simulink model "dts_adc1"  (R2023b)
settings: Solver=VariableStepAuto  StartTime=0.0  StopTime=3*DF/Fs  MaxStep=10/12e6  MinStep=1/12e6  RelTol=1e-9  AbsTol=1e-9  EnableMultiTasking=on
model workspace (MAT data in the model file):
  Q = 1.6e-19
  k = 1.38e-23
  m = 4
  p = 8
values from neighbouring files (symbols this model uses):
  a = 4.32    [ADC_data2.m]    (also in ADC_filter_data.mat)
  DF = 512    [ADC_data2.m]    (also in ADC_filter_data.mat)
  Fs = 1e+06    (= 1000000)    [ADC_data2.m]    (also in ADC_filter_data.mat)
  T = temp + 273.15    [ADC_data2.m]    (also in ADC_filter_data.mat = 428.15)
  vctat = -VCTAT(i)    [ADC_data2.m]    (also in ADC_filter_data.mat = -0.648)
  vn = 10e-6    (= 1e-05)    [ADC_data2.m]    (also in ADC_filter_data.mat)
  vos = 0    [ADC_data2.m]    (also in ADC_filter_data.mat)
  vptat = VPTAT(i)    [ADC_data2.m]    (also in ADC_filter_data.mat = 0.692)
undefined symbols (not defined in the file or in its folder): Nsamples, OSR
libraries: dspstat3 x2, dspsigops x2
settings Model: Creator=amyles  LastModifiedBy=SinhaAd
settings SolverCC: InitialStep=0  AlgebraicLoopSolver=TrustRegion
settings DataIOCC: LimitDataPoints=on  MaxDataPoints=50000  SaveFormat=Array  ReturnWorkspaceOutputs=off  Refine=10
settings OptimizationCC: DefaultParameterBehavior=Inlined  ExpressionDepthLimit=2147483647  LifeSpan=inf
settings DebuggingCC: SolverPrmCheckMsg=warning  FcnCallInpInsideContextMsg=warning  UnconnectedInputMsg=warning  UnconnectedOutputMsg=warning  UnconnectedLineMsg=warning  StateNameClashWarn=warning  StrictBusMsg=ErrorOnBusTreatedAsVector  SFUnexpectedBacktrackingDiag=warning  SFNoUnconditionalDefaultTransitionDiag=warning  SFExecutionAtInitializationDiag=none  ArithmeticOperatorsInVariantConditions=warning
settings HardwareCC: ProdBitPerPointer=32  ProdBitPerSizeT=32  ProdBitPerPtrDiffT=32  ProdLargestAtomicFloat=None  ProdIntDivRoundTo=Undefined  ProdEndianess=Unspecified  ProdWordSize=32  ProdHWDeviceType=32-bit Generic
settings ModelReferenceCC: EnableRefExpFcnMdlSchedulingChecks=on  ModelReferenceNumInstancesAllowed=Single  PropagateSignalLabelsOutOfModel=off
settings SFSimCC: SimUseLocalCustomCode=off  CustomCodeUndefinedFunction=UseInterfaceOnly
settings RTWCC: RTWUseLocalCustomCode=off  DLArmComputeVersion=19.05
settings CodeAppCC: StateflowObjectComments=on
settings GRTTargetCC: TargetLangStandard=C89/C90 (ANSI)  CombineOutputUpdateFcns=off  GRTInterface=on
settings ConfigComp: CovMetricSettings=dw  CovSaveCumulativeToWorkspaceVar=on  CovSaveSingleToWorkspaceVar=on  CovExternalEMLEnable=off

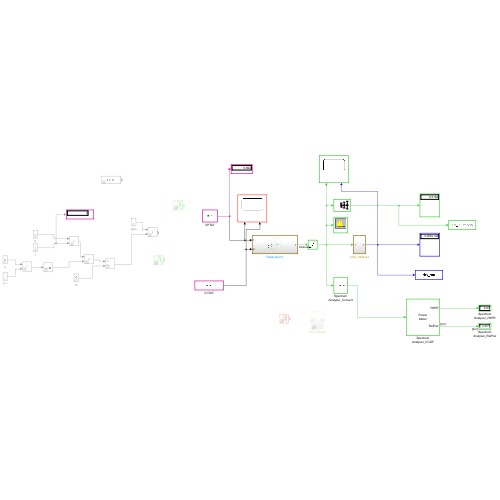
[thumbnail: Simulink's stored preview of the top-level diagram]
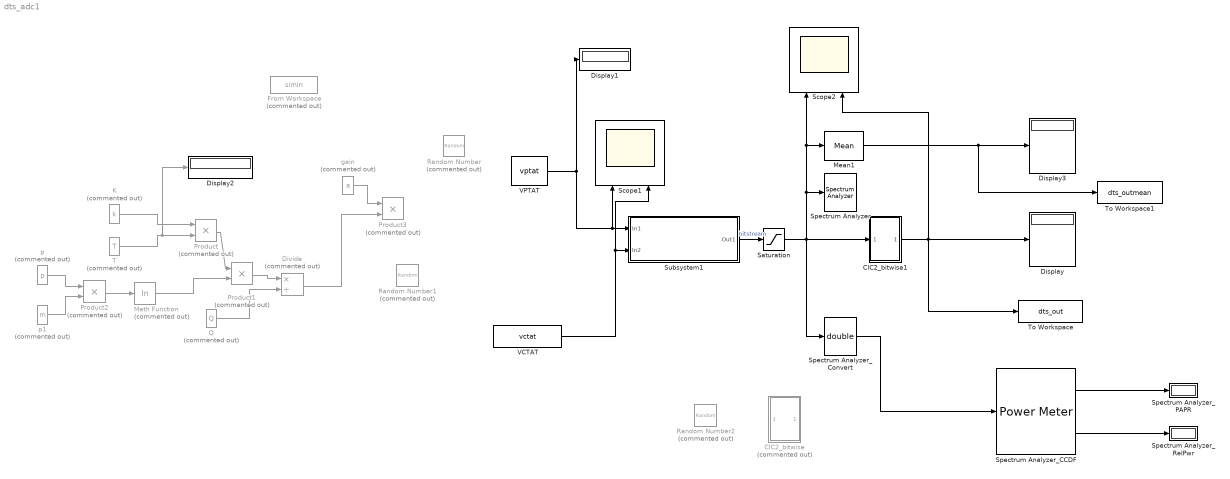
== system dts_adc1 ==
  CIC2_bitwise : Subsystem  Commented=on
  CIC2_bitwise1 : Subsystem
  Display{,1..3} (4 alike) : Display
  Divide : Product  Commented=on  Inputs=*/
  From Workspace : FromWorkspace  Commented=on  VariableName=simin
  K : Constant  Commented=on  Value=k
  Math Function : Math  Commented=on  Operator=log
  Mean1 : dspstat3/Mean  run=on  reset_popup=None  directionMode=Entire input  dimension=1  roiEnable=off  roiType=Rectangles  roiPortion=Entire ROI  roiOutput=Individual statistics for each ROI  roiFlag=off  roundingMode=Floor  overflowMode=off  outputDataTypeStr=Inherit: Same as accumulator  outputMin=[]  outputMax=[]  outputLastDataTypeStr=Inherit: Same as accumulator
  Product{,1..3} (4 alike) : Product  Commented=on
  Q : Constant  Commented=on  Value=Q
  Random Number : RandomNumber  Commented=on  Variance=(vn)^2  Seed=12345  SampleTime=1/(10*Fs)
  Random Number1 : RandomNumber  Commented=on  Variance=(vn)^2  SampleTime=1/(10*Fs)
  Random Number2 : RandomNumber  Commented=on  Variance=(1e-3)^2  SampleTime=1/(10*Fs)
  Saturation : Saturate  UpperLimit=1  LowerLimit=0
  Scope1 : Scope  NumInputPorts=2
  Scope2 : Scope  NumInputPorts=2
  Spectrum Analyzer : SpectrumAnalyzer  WindowPosition=[196.000000,277.000000,1278.000000,670.000000,]  Visible=on  ScopeFrameLocation=window  Method=Welch  SampleRateSource=Property  SampleRate=Fs  PlotAsTwoSidedSpectrum=off  FrequencyScale=Log  AveragingMethod=Exponential  YLimits=[-62.38980233,33.88782663]  SelectedToolstripTab=spectrumAnalyzerToolstrip.measurementsTab  DefaultConfigurationName=spbscopes.SpectrumAnalyzerBlockCfg  IsFrequencyInputMode=0  FrequencyVectorPort=0  FrequencyVectorFromPort=0  FrequencyInputRBWPort=0  FrequencyInputRBWFromPort=0
  Spectrum Analyzer_CCDF : dspstat3/Power Meter  Measurement=Peak-to-average power ratio  ReferenceLoad=1  OutputPowerUnits=dBm  WindowLength=256  OverlapLength=255  AllowArbitraryInputLength=off  ComputeCCDF=on  PowerRange=50  PowerResolution=0.1  CCDFOutput=Relative power (dB above average power)  ProbabilityVector=[ 10; 1; 0.1; 0.01; 0.001; 0.0001 ]  RelativePowerVector=[ 0; 3; 6; 9; 12 ]  ResetPort=off  SimulateUsing=Code generation
  Spectrum Analyzer_Convert : DataTypeConversion  OutDataTypeStr=double
  Spectrum Analyzer_PAPR : Display
  Spectrum Analyzer_RelPwr : Display
  Subsystem1 : Subsystem
  T : Constant  Commented=on  Value=T
  To Workspace : ToWorkspace  VariableName=dts_out  SaveFormat=Timeseries  SampleTime=-1
  To Workspace1 : ToWorkspace  VariableName=dts_outmean  SaveFormat=Timeseries  SampleTime=-1
  VCTAT : Constant  Value=vctat
  VPTAT : Constant  Value=vptat
  gain : Constant  Commented=on  Value=a
  p : Constant  Commented=on  Value=p
  p1 : Constant  Commented=on  Value=m
  wires:
  VPTAT/1 -> Scope1/1, Subsystem1/1(In1), Display1/1
  Subsystem1/1(Out1) -> Saturation/1  "bitstream"
  K/1 -> Product/1
  T/1 -> Display2/1, Product/2
  Q/1 -> Divide/2
  Product/1 -> Product1/1
  Product1/1 -> Divide/1
  Product2/1 -> Math Function/1
  p/1 -> Product2/1
  p1/1 -> Product2/2
  Math Function/1 -> Product1/2
  Divide/1 -> Product3/2
  gain/1 -> Product3/1
  Saturation/1 -> Spectrum Analyzer_Convert/1, Spectrum Analyzer/1, Mean1/1, Scope2/1, CIC2_bitwise1/1(In1)
  CIC2_bitwise1/1(Outport) -> Scope2/2, To Workspace/1, Display/1
  VCTAT/1 -> Scope1/2, Subsystem1/2(In2)
  Spectrum Analyzer_Convert/1 -> Spectrum Analyzer_CCDF/1
  Spectrum Analyzer_CCDF/1 -> Spectrum Analyzer_PAPR/1
  Spectrum Analyzer_CCDF/2 -> Spectrum Analyzer_RelPwr/1
  Mean1/1 -> To Workspace1/1, Display3/1

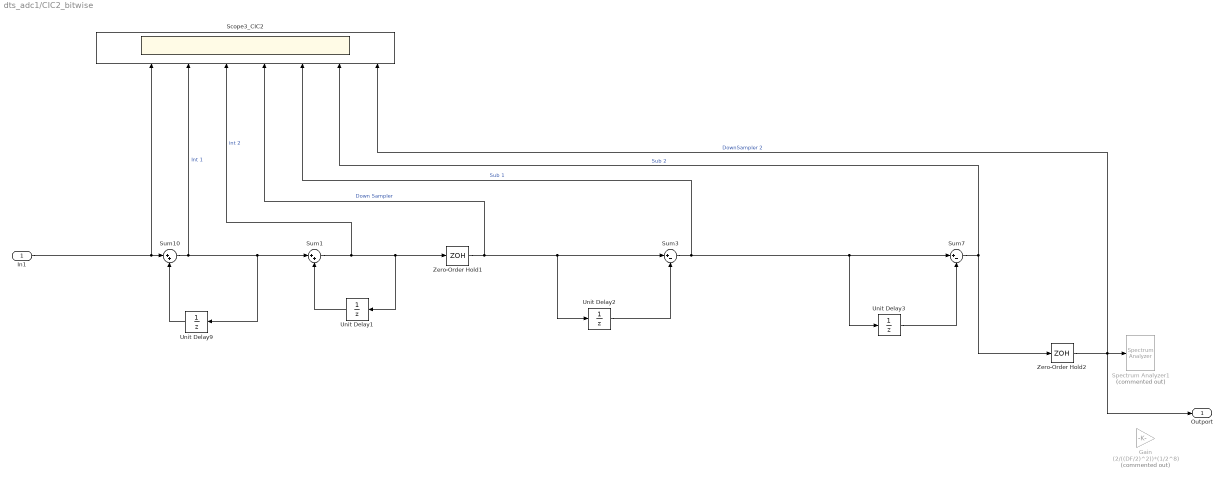
== system dts_adc1/CIC2_bitwise ==
  In1 : Inport
  Gain : Gain  Commented=on  Gain=(2/((DF/2)^2))*(1/2^8)
  Scope3_CIC2 : Scope  NumInputPorts=8
  Spectrum Analyzer1 : SpectrumAnalyzer  Commented=on  WindowPosition=[1.8 41.8 1534.4 740.8]  Method=Welch  SampleRate=5859.375  PlotAsTwoSidedSpectrum=off  AxesScaling=Manual  FrequencySpan=Start and stop frequencies  Span=(2*16*12e6)/2048  StartFrequency=0.9  StopFrequency=Fs/(2*32*OSR)  FrequencyResolutionMethod=Window length  WindowLength=(Nsamples)/(OSR)  AveragingMethod=Exponential  YLimits=[-39.824711379585536974,154.79966114651364251]  ShowLegend=on  DefaultConfigurationName=spbscopes.SpectrumAnalyzerBlockCfg  IsFrequencyInputMode=0  FrequencyVectorPort=0  FrequencyVectorFromPort=0  FrequencyInputRBWPort=0  FrequencyInputRBWFromPort=0
  Sum1 : Sum  Inputs=|++  OutDataTypeStr=fixdt(1,35,0)  AccumDataTypeStr=fixdt(1,35,0)  SaturateOnIntegerOverflow=on
  Sum10 : Sum  Inputs=|++  OutDataTypeStr=fixdt(1,22,0)  AccumDataTypeStr=fixdt(1,22,0)  SaturateOnIntegerOverflow=on
  Sum3 : Sum  Inputs=|+-  OutDataTypeStr=fixdt(1,35,0)  AccumDataTypeStr=fixdt(1,35,0)  SaturateOnIntegerOverflow=on
  Sum7 : Sum  Inputs=|+-  OutDataTypeStr=fixdt(1,35,0)  AccumDataTypeStr=fixdt(1,35,0)  SaturateOnIntegerOverflow=on
  Unit Delay1 : UnitDelay  SampleTime=1/Fs  HasFrameUpgradeWarning=on
  Unit Delay2 : UnitDelay  SampleTime=DF/(2*Fs)  HasFrameUpgradeWarning=on
  Unit Delay3 : UnitDelay  SampleTime=DF/(2*Fs)  HasFrameUpgradeWarning=on
  Unit Delay9 : UnitDelay  SampleTime=1/Fs  HasFrameUpgradeWarning=on
  Zero-Order Hold1 : ZeroOrderHold  SampleTime=(DF)/(2*Fs)
  Zero-Order Hold2 : ZeroOrderHold  SampleTime=(DF)/(Fs)
  Outport : Outport
  wires:
  Sum1/1 -> Unit Delay1/1, Zero-Order Hold1/1, Scope3_CIC2/4  "int 2"
  Sum3/1 -> Unit Delay3/1, Sum7/1, Scope3_CIC2/6  "Sub 1"
  Sum10/1 -> Unit Delay9/1, Sum1/1, Scope3_CIC2/3  "Int 1"
  Zero-Order Hold1/1 -> Scope3_CIC2/5, Unit Delay2/1, Sum3/1  "Down Sampler"
  In1/1 -> Scope3_CIC2/2, Sum10/1
  Unit Delay3/1 -> Sum7/2
  Unit Delay9/1 -> Sum10/2
  Unit Delay2/1 -> Sum3/2
  Sum7/1 -> Scope3_CIC2/7, Zero-Order Hold2/1  "Sub 2"
  Zero-Order Hold2/1 -> Outport/1, Scope3_CIC2/8, Spectrum Analyzer1/1  "DownSampler 2"
  Unit Delay1/1 -> Sum1/2

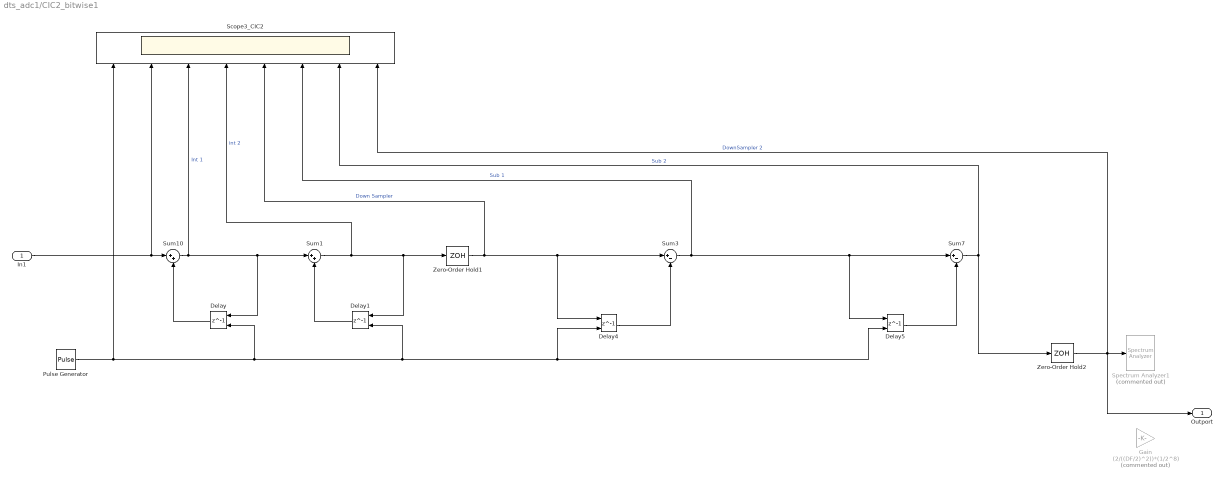
== system dts_adc1/CIC2_bitwise1 ==
  In1 : Inport
  Delay : Delay  DelayLength=1  ExternalReset=Rising  SampleTime=1/Fs
      settings: InputPortMap=u0,r5
  Delay1 : Delay  DelayLength=1  ExternalReset=Rising  SampleTime=1/Fs
      settings: InputPortMap=u0,r5
  Delay4 : Delay  DelayLength=1  ExternalReset=Rising  SampleTime=(DF)/(2*Fs)
      settings: InputPortMap=u0,r5
  Delay5 : Delay  DelayLength=1  ExternalReset=Rising  SampleTime=(DF)/(2*Fs)
      settings: InputPortMap=u0,r5
  Gain : Gain  Commented=on  Gain=(2/((DF/2)^2))*(1/2^8)
  Pulse Generator : DiscretePulseGenerator  PulseType=Time based  Period=4*DF/Fs  PulseWidth=50  PhaseDelay=0.5/Fs
  Scope3_CIC2 : Scope  NumInputPorts=8
  Spectrum Analyzer1 : SpectrumAnalyzer  Commented=on  WindowPosition=[1.8 41.8 1534.4 740.8]  Method=Welch  SampleRate=5859.375  PlotAsTwoSidedSpectrum=off  AxesScaling=Manual  FrequencySpan=Start and stop frequencies  Span=(2*16*12e6)/2048  StartFrequency=0.9  StopFrequency=Fs/(2*32*OSR)  FrequencyResolutionMethod=Window length  WindowLength=(Nsamples)/(OSR)  AveragingMethod=Exponential  YLimits=[-39.824711379585536974,154.79966114651364251]  ShowLegend=on  DefaultConfigurationName=spbscopes.SpectrumAnalyzerBlockCfg  IsFrequencyInputMode=0  FrequencyVectorPort=0  FrequencyVectorFromPort=0  FrequencyInputRBWPort=0  FrequencyInputRBWFromPort=0
  Sum1 : Sum  Inputs=|++  OutDataTypeStr=fixdt(1,32,0)  AccumDataTypeStr=fixdt(1,32,0)  SaturateOnIntegerOverflow=on
  Sum10 : Sum  Inputs=|++  OutDataTypeStr=fixdt(1,32,0)  AccumDataTypeStr=fixdt(1,32,0)  SaturateOnIntegerOverflow=on
  Sum3 : Sum  Inputs=|+-  OutDataTypeStr=fixdt(1,32,0)  AccumDataTypeStr=fixdt(1,32,0)  SaturateOnIntegerOverflow=on
  Sum7 : Sum  Inputs=|+-  OutDataTypeStr=fixdt(1,32,0)  AccumDataTypeStr=fixdt(1,32,0)  SaturateOnIntegerOverflow=on
  Zero-Order Hold1 : ZeroOrderHold  SampleTime=(DF)/(2*Fs)
  Zero-Order Hold2 : ZeroOrderHold  SampleTime=(DF)/(Fs)
  Outport : Outport
  wires:
  Sum1/1 -> Zero-Order Hold1/1, Delay1/1, Scope3_CIC2/4  "int 2"
  Sum3/1 -> Delay5/1, Sum7/1, Scope3_CIC2/6  "Sub 1"
  Sum10/1 -> Scope3_CIC2/3, Delay/1, Sum1/1  "Int 1"
  Zero-Order Hold1/1 -> Scope3_CIC2/5, Delay4/1, Sum3/1  "Down Sampler"
  In1/1 -> Scope3_CIC2/2, Sum10/1
  Delay5/1 -> Sum7/2
  Delay1/1 -> Sum1/2
  Delay/1 -> Sum10/2
  Delay4/1 -> Sum3/2
  Pulse Generator/1 -> Scope3_CIC2/1, Delay/2, Delay1/2, Delay4/2, Delay5/2
  Sum7/1 -> Scope3_CIC2/7, Zero-Order Hold2/1  "Sub 2"
  Zero-Order Hold2/1 -> Outport/1, Scope3_CIC2/8, Spectrum Analyzer1/1  "DownSampler 2"

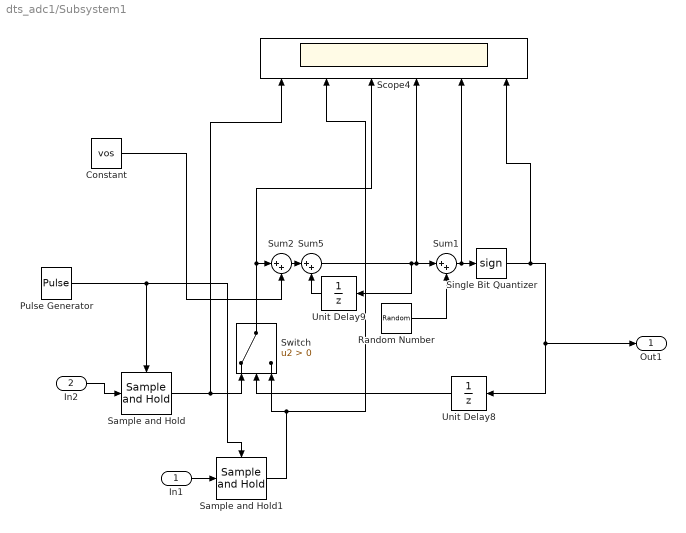
== system dts_adc1/Subsystem1 ==
  In1 : Inport
  In2 : Inport  Port=2
  Constant : Constant  Value=vos
  Pulse Generator : DiscretePulseGenerator  PulseType=Time based  Period=1/Fs  PulseWidth=50
  Random Number : RandomNumber  Variance=(50e-3)^2  SampleTime=1/Fs
  Sample and Hold : dspsigops/Sample and Hold  trig=Rising edge  initCond=0  latchinput=off
  Sample and Hold1 : dspsigops/Sample and Hold  trig=Rising edge  initCond=0  latchinput=off
  Scope4 : Scope  NumInputPorts=6
  Single Bit Quantizer : Signum  SampleTime=1/Fs
  Sum1 : Sum  Inputs=|++
  Sum2 : Sum  Inputs=|++
  Sum5 : Sum  Inputs=|++
  Switch : Switch  Criteria=u2 > Threshold  SaturateOnIntegerOverflow=off  InputSameDT=off
  Unit Delay8 : UnitDelay  SampleTime=1/Fs  HasFrameUpgradeWarning=on
  Unit Delay9 : UnitDelay  SampleTime=1/Fs  HasFrameUpgradeWarning=on
  Out1 : Outport
  wires:
  Sum1/1 -> Scope4/5, Single Bit Quantizer/1
  Unit Delay9/1 -> Sum5/2
  Sum5/1 -> Scope4/4, Sum1/1, Unit Delay9/1
  Random Number/1 -> Sum1/2
  Single Bit Quantizer/1 -> Out1/1, Unit Delay8/1, Scope4/6
  Switch/1 -> Scope4/3, Sum2/1
  Unit Delay8/1 -> Switch/2
  In2/1 -> Sample and Hold/1
  In1/1 -> Sample and Hold1/1
  Sample and Hold/1 -> Switch/1, Scope4/1
  Sample and Hold1/1 -> Scope4/2, Switch/3
  Pulse Generator/1 -> Sample and Hold1/Trigger, Sample and Hold/Trigger
  Sum2/1 -> Sum5/1
  Constant/1 -> Sum2/2
